simulink model "BSCU_Active_State"  (Simulink 8.7)
settings: Solver=VariableStepAuto  StartTime=0.0  StopTime=10.0  RelTol=1e-3
settings Model: Creator=bourbouh  LastModifiedBy=bourbouh
settings DataIOCC: LimitDataPoints=off  SaveFormat=Dataset
settings DebuggingCC: UnderspecifiedInitializationDetection=Simplified  MergeDetectMultiDrivingBlocksExec=error
settings HardwareCC: ProdBitPerPointer=64  ProdLargestAtomicFloat=Float  ProdIntDivRoundTo=Zero  ProdEndianess=LittleEndian  ProdWordSize=64  ProdHWDeviceType=Intel->x86-64 (Windows64)
settings ModelReferenceCC: PropagateSignalLabelsOutOfModel=on
settings ConfigComp: CovModelRefEnable=off

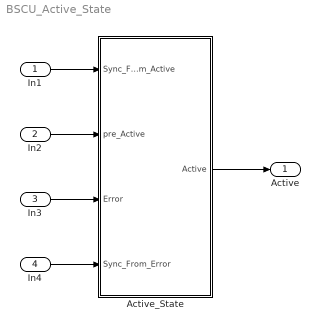
== system BSCU_Active_State ==
  In1 : Inport
  In2 : Inport  Port=2
  In3 : Inport  Port=3
  In4 : Inport  Port=4
  Active_State : Stateflow chart  TreatAsAtomicUnit=on
  Active : Outport
  wires:
  In1/1 -> Active_State/1(Sync_From_Active)
  In2/1 -> Active_State/2(pre_Active)
  In3/1 -> Active_State/3(Error)
  In4/1 -> Active_State/4(Sync_From_Error)
  Active_State/1(Active) -> Active/1

== stateflow chart Active_State ==
  (default) -> (junction 9)
  (junction 9) -> (junction 10) [order 1] : [Error]
  (junction 9) -> (junction 11) [order 2]
  (junction 10) -> (junction 18) : {Active = false;}
  (junction 11) -> (junction 12) [order 1] : [pre_Active && Sync_From_Active && (! Sync_From_Error) && (! Primary_Side) ]
  (junction 11) -> (junction 13) [order 2]
  (junction 12) -> (junction 17) : {Active = false;}
  (junction 13) -> (junction 14) [order 1] : [(!pre_Active) && ( (!Sync_From_Active) || Sync_From_Error)]
  (junction 13) -> (junction 15) [order 2] : {Active = pre_Active;}
  (junction 14) -> (junction 16) : {Active = true;}
  (junction 16) -> (junction 15)
  (junction 17) -> (junction 16)
  (junction 18) -> (junction 17)
  (junction 15) -> (junction 19)
  data: Sync_From_Active input boolean; Active output boolean; pre_Active input boolean; Error input boolean; Sync_From_Error input boolean; Primary_Side parameter double
